simulink model "q4sl"  (R2025b)
settings: Solver=VariableStepAuto  StartTime=0.0  StopTime=10.0  RelTol=1e-3
undefined symbols (not defined in the file or in its folder): stepp
settings Model: Creator=Qi Zhang  LastModifiedBy=Qi Zhang

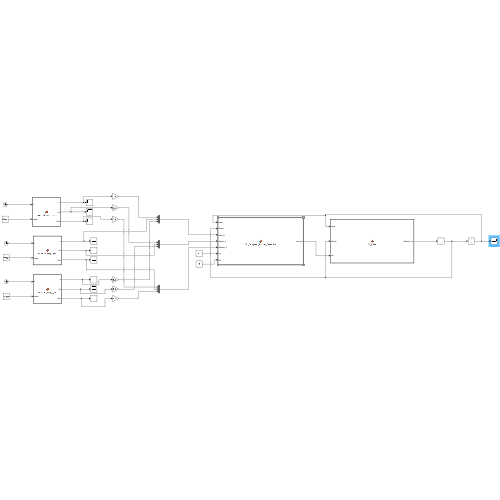
[thumbnail: Simulink's stored preview of the top-level diagram]
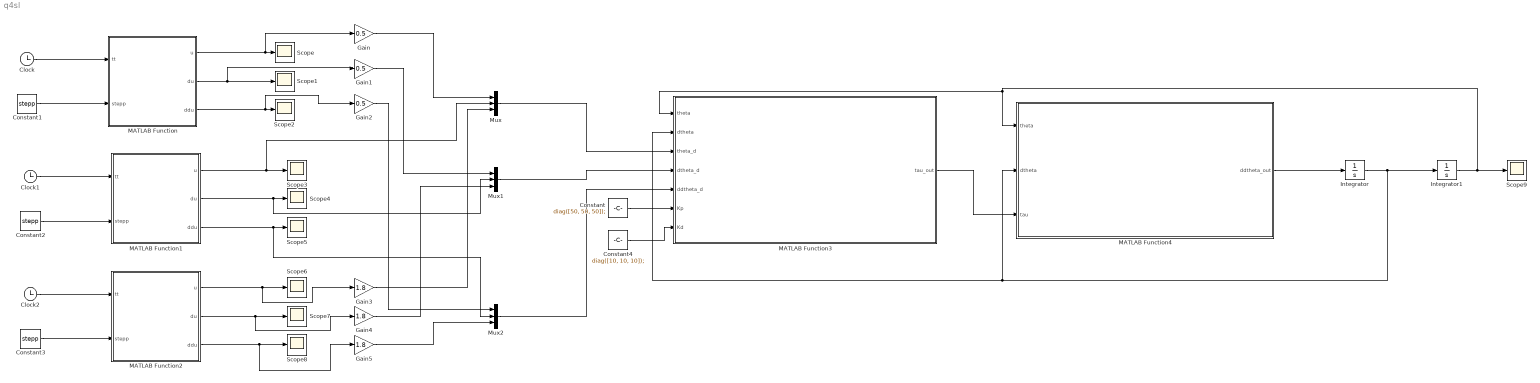
== system q4sl ==
  Clock : Clock
  Clock1 : Clock
  Clock2 : Clock
  Constant : Constant  Value=diag([50, 50, 50]);
  Constant1 : Constant  Value=stepp
  Constant2 : Constant  Value=stepp
  Constant3 : Constant  Value=stepp
  Constant4 : Constant  Value=diag([10, 10, 10]);
  Gain : Gain  Gain=0.5
  Gain1 : Gain  Gain=0.5
  Gain2 : Gain  Gain=0.5
  Gain3 : Gain  Gain=1.8
  Gain4 : Gain  Gain=1.8
  Gain5 : Gain  Gain=1.8
  Integrator : Integrator  InitialCondition=[0;0;0]
  Integrator1 : Integrator  InitialCondition=[0;0;0]
  MATLAB Function : MATLAB Function  TreatAsAtomicUnit=on
  MATLAB Function1 : MATLAB Function  TreatAsAtomicUnit=on
  MATLAB Function2 : MATLAB Function  TreatAsAtomicUnit=on
  MATLAB Function3 : MATLAB Function  TreatAsAtomicUnit=on
  MATLAB Function4 : MATLAB Function  TreatAsAtomicUnit=on
  Mux : Mux  Inputs=3
  Mux1 : Mux  Inputs=3
  Mux2 : Mux  Inputs=3
  Scope{,1..9} (10 alike) : Scope
      Scope settings: ActiveDisplayYMinimum=-1  ActiveDisplayYMaximum=1
      Scope1 settings: ActiveDisplayYMinimum=-0.071428571428571411  ActiveDisplayYMaximum=0.64285714285714279
      Scope2 settings: ActiveDisplayYMinimum=-2.8571428571428568  ActiveDisplayYMaximum=2.8571428571428568  DataLoggingVariableName=ScopeData2
      Scope3 settings: ActiveDisplayYMinimum=-0.12499999999999997  ActiveDisplayYMaximum=1.125  DataLoggingVariableName=ScopeData3
      Scope4 settings: ActiveDisplayYMinimum=-0.071428571428571411  ActiveDisplayYMaximum=0.64285714285714279  DataLoggingVariableName=ScopeData4
      Scope5 settings: ActiveDisplayYMinimum=-2.8571428571428568  ActiveDisplayYMaximum=2.8571428571428568  DataLoggingVariableName=ScopeData5
      Scope6 settings: ActiveDisplayYMinimum=-0.12499999999999997  ActiveDisplayYMaximum=1.125  DataLoggingVariableName=ScopeData6
      Scope7 settings: ActiveDisplayYMinimum=-0.071428571428571411  ActiveDisplayYMaximum=0.64285714285714279  DataLoggingVariableName=ScopeData7
      Scope8 settings: ActiveDisplayYMinimum=-2.8571428571428568  ActiveDisplayYMaximum=2.8571428571428568  DataLoggingVariableName=ScopeData8
      Scope9 settings: ActiveDisplayYMinimum=-0.22616549126415639  ActiveDisplayYMaximum=2.0354894213774082  DataLoggingVariableName=ScopeData9
  wires:
  Gain/1 -> Mux/1
  Gain3/1 -> Mux/3
  Gain4/1 -> Mux1/3
  Gain1/1 -> Mux1/1
  Gain5/1 -> Mux2/3
  Clock2/1 -> MATLAB Function2/1(tt)
  MATLAB Function2/3(ddu) -> Gain5/1, Scope8/1
  MATLAB Function2/1(u) -> Gain3/1, Scope6/1
  Mux2/1 -> MATLAB Function3/5(ddtheta_d)
  MATLAB Function2/2(du) -> Gain4/1, Scope7/1
  MATLAB Function1/3(ddu) -> Mux2/2, Scope5/1
  MATLAB Function1/2(du) -> Mux1/2, Scope4/1
  Constant2/1 -> MATLAB Function1/2(stepp)
  Clock1/1 -> MATLAB Function1/1(tt)
  MATLAB Function/3(ddu) -> Gain2/1, Scope2/1
  Clock/1 -> MATLAB Function/1(tt)
  MATLAB Function/1(u) -> Gain/1, Scope/1
  Constant1/1 -> MATLAB Function/2(stepp)
  MATLAB Function1/1(u) -> Mux/2, Scope3/1
  Constant3/1 -> MATLAB Function2/2(stepp)
  MATLAB Function/2(du) -> Scope1/1, Gain1/1
  Gain2/1 -> Mux2/1
  MATLAB Function3/1(tau_out) -> MATLAB Function4/3(tau)
  MATLAB Function4/1(ddtheta_out) -> Integrator/1
  Integrator/1 -> MATLAB Function4/2(dtheta), MATLAB Function3/2(dtheta), Integrator1/1
  Integrator1/1 -> Scope9/1, MATLAB Function3/1(theta), MATLAB Function4/1(theta)
  Mux/1 -> MATLAB Function3/3(theta_d)
  Mux1/1 -> MATLAB Function3/4(dtheta_d)
  Constant/1 -> MATLAB Function3/6(Kp)
  Constant4/1 -> MATLAB Function3/7(Kd)

== matlab function q4sl/MATLAB Function1 ==
  data: tt input; u output; stepp input; du output; ddu output
function [u,du,ddu] = rounded_step_gen(tt,stepp)
    %{
    Three input parameters are passed to this function in the
    list stepp, namely st0, t1 and t3, in this sequence.
    
    Function to generate a rounded unit step function of time, tt.
    If st0 is zero, the step is generated as starting with zero
    slope at time 0 and increasing with a parabolic curve until t1.
    Then it changes to increasing linearly with the same slope as
    that of the parabola at t1, until t2 (which is calculated by
    the function), after which it increases with negative second
    derivative, with the same parabolic shape, until it reaches the
    unit step function value at t3, with zero slope.  The slope of
    the curve is the same just before and just after t2.

    The whole rounded step can be delayed by st0.    
    %}
    st0 = stepp(1);t1 = stepp(2);t3 = stepp(3);
    alpha = 1/(t3 - t1)/t1/2;
    beta  = -alpha*t1*t1;
    t2    = t3 - t1;

    A = [t2, 1;t3, 1];
    b = [alpha*(t2*t2 + 2*t1*t2 - t1*t1);1 + alpha*t3*t3];

    x = A\b;
    gamma = x(1);
    eta   = x(2);

    st1 = st0 + t1;
    st2 = st0 + t2;
    st3 = st0 + t3;
    ta  = tt - st0;
    if tt <= st0
        u   = 0;
        du  = 0;
        ddu = 0;
    elseif tt <= st1
        u   = alpha*ta*ta;
        ddu = 2*alpha;
        du  = ddu*ta;
    elseif tt <= st2
        u   = 2*alpha*t1*ta + beta;
        du  = 2*alpha*t1;
        ddu = 0;
    elseif tt <= st3
        u   = -alpha*ta*ta + gamma*ta + eta;
        ddu = -2*alpha;
        du  = ddu*ta + gamma;
    else
        u  = 1;
        du  = 0;
        ddu = 0;
    end
end

== matlab function q4sl/MATLAB Function ==
  data: tt input; u output; stepp input; du output; ddu output
function [u,du,ddu] = rounded_step_gen(tt,stepp)
    %{
    Three input parameters are passed to this function in the
    list stepp, namely st0, t1 and t3, in this sequence.
    
    Function to generate a rounded unit step function of time, tt.
    If st0 is zero, the step is generated as starting with zero
    slope at time 0 and increasing with a parabolic curve until t1.
    Then it changes to increasing linearly with the same slope as
    that of the parabola at t1, until t2 (which is calculated by
    the function), after which it increases with negative second
    derivative, with the same parabolic shape, until it reaches the
    unit step function value at t3, with zero slope.  The slope of
    the curve is the same just before and just after t2.

    The whole rounded step can be delayed by st0.    
    %}
    st0 = stepp(1);t1 = stepp(2);t3 = stepp(3);
    alpha = 1/(t3 - t1)/t1/2;
    beta  = -alpha*t1*t1;
    t2    = t3 - t1;

    A = [t2, 1;t3, 1];
    b = [alpha*(t2*t2 + 2*t1*t2 - t1*t1);1 + alpha*t3*t3];

    x = A\b;
    gamma = x(1);
    eta   = x(2);

    st1 = st0 + t1;
    st2 = st0 + t2;
    st3 = st0 + t3;
    ta  = tt - st0;
    if tt <= st0
        u   = 0;
        du  = 0;
        ddu = 0;
    elseif tt <= st1
        u   = alpha*ta*ta;
        ddu = 2*alpha;
        du  = ddu*ta;
    elseif tt <= st2
        u   = 2*alpha*t1*ta + beta;
        du  = 2*alpha*t1;
        ddu = 0;
    elseif tt <= st3
        u   = -alpha*ta*ta + gamma*ta + eta;
        ddu = -2*alpha;
        du  = ddu*ta + gamma;
    else
        u  = 1;
        du  = 0;
        ddu = 0;
    end
end

== matlab function q4sl/MATLAB Function2 ==
  data: tt input; u output; stepp input; du output; ddu output
function [u,du,ddu] = rounded_step_gen(tt,stepp)
    %{
    Three input parameters are passed to this function in the
    list stepp, namely st0, t1 and t3, in this sequence.
    
    Function to generate a rounded unit step function of time, tt.
    If st0 is zero, the step is generated as starting with zero
    slope at time 0 and increasing with a parabolic curve until t1.
    Then it changes to increasing linearly with the same slope as
    that of the parabola at t1, until t2 (which is calculated by
    the function), after which it increases with negative second
    derivative, with the same parabolic shape, until it reaches the
    unit step function value at t3, with zero slope.  The slope of
    the curve is the same just before and just after t2.

    The whole rounded step can be delayed by st0.    
    %}
    st0 = stepp(1);t1 = stepp(2);t3 = stepp(3);
    alpha = 1/(t3 - t1)/t1/2;
    beta  = -alpha*t1*t1;
    t2    = t3 - t1;

    A = [t2, 1;t3, 1];
    b = [alpha*(t2*t2 + 2*t1*t2 - t1*t1);1 + alpha*t3*t3];

    x = A\b;
    gamma = x(1);
    eta   = x(2);

    st1 = st0 + t1;
    st2 = st0 + t2;
    st3 = st0 + t3;
    ta  = tt - st0;
    if tt <= st0
        u   = 0;
        du  = 0;
        ddu = 0;
    elseif tt <= st1
        u   = alpha*ta*ta;
        ddu = 2*alpha;
        du  = ddu*ta;
    elseif tt <= st2
        u   = 2*alpha*t1*ta + beta;
        du  = 2*alpha*t1;
        ddu = 0;
    elseif tt <= st3
        u   = -alpha*ta*ta + gamma*ta + eta;
        ddu = -2*alpha;
        du  = ddu*ta + gamma;
    else
        u  = 1;
        du  = 0;
        ddu = 0;
    end
end

== matlab function q4sl/MATLAB Function3 ==
  data: theta input; tau_out output; dtheta input; theta_d input; dtheta_d input; ddtheta_d input; Kp input; Kd input
function tau_out = SL_Compute_Torque_Controller(theta, dtheta, theta_d, dtheta_d, ddtheta_d, Kp, Kd)

% theta     = reshape(theta,     [4,1]);
% dtheta    = reshape(dtheta,    [4,1]);
% theta_d   = reshape(theta_d,   [4,1]);
% dtheta_d  = reshape(dtheta_d,  [4,1]);
% ddtheta_d = reshape(ddtheta_d, [4,1]);

% Kp = reshape(Kp, [4,4]);
% Kd = reshape(Kd, [4,4]);

% M = zeros(4,4);
% C = zeros(4,4);
% N = zeros(4,1);

M = calc_M_25_b(theta);
C = calc_C_25_b(theta, dtheta);
N = calc_N_25_b(theta, dtheta);

e  = theta_d - theta;
de = dtheta_d - dtheta;

v = ddtheta_d + Kd*de + Kp*e;

% tau_out = zeros(4,1);
tau_out = M*v + C*dtheta + N;

end

== matlab function q4sl/MATLAB Function4 ==
  data: theta input; ddtheta_out output; dtheta input; tau input
function ddtheta_out = SL_Plant(theta, dtheta, tau)


% theta  = reshape(theta,  [4,1]);
% dtheta = reshape(dtheta, [4,1]);
% tau    = reshape(tau,    [4,1]);

% M = zeros(4,4);
% C = zeros(4,4);
% N = zeros(4,1);

M = calc_M_25_b(theta);
C = calc_C_25_b(theta, dtheta);
N   = calc_N_25_b(theta, dtheta);

% rhs = zeros(4,1);
rhs = tau - C*dtheta - N;

% ddtheta_out = zeros(4,1);
ddtheta_out = M \ rhs;
end
